simulink model "Lab3Part2B2"  (R2025b)
settings: Solver=VariableStepAuto  StartTime=0.0  StopTime=10.0  RelTol=1e-3
values from neighbouring files (symbols this model uses):
  A = [0 0 1 0 ... (first row only)    [Lab3Part2B1.m]
  B = [0 ... (first row only)    [Lab3Part2B1.m]
  K = place(A,B,desired_poles)    [Lab3Part2B1.m]
libraries: simulink_extras x3
settings Model: Creator=safiakhalil  LastModifiedBy=safiakhalil

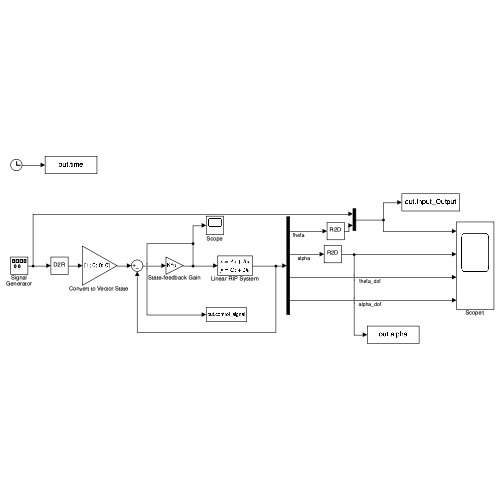
[thumbnail: Simulink's stored preview of the top-level diagram]
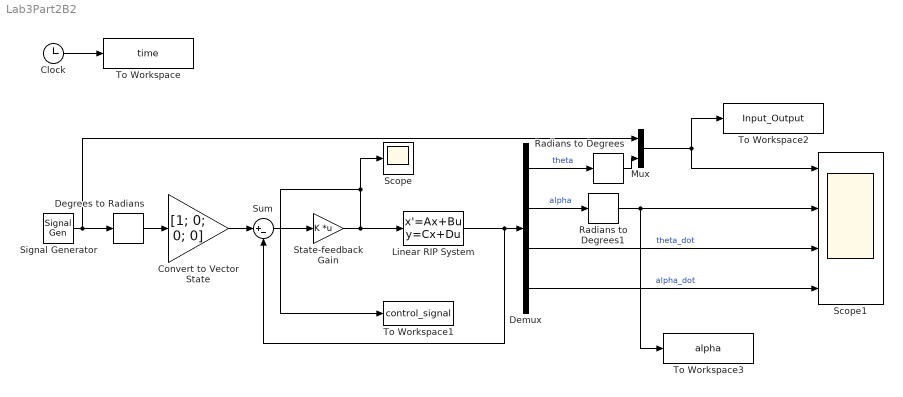
== system Lab3Part2B2 ==
  Clock : Clock
  "Convert to Vector State " : Gain  Gain=[1; 0; 0; 0]
  Degrees to Radians : simulink_extras/Transformations/Degrees to Radians
  Demux : Demux
  Linear RIP System : StateSpace  A=A  B=B  C=eye(4)  D=zeros(4, 1)  InitialCondition=0
  Mux : Mux  Inputs=2
  Radians to Degrees : simulink_extras/Transformations/Radians to Degrees
  Radians to Degrees1 : simulink_extras/Transformations/Radians to Degrees
  Scope : Scope
      settings: ActiveDisplayYMinimum=-0.48303961854114436  ActiveDisplayYMaximum=0.48467023948413279
  Scope1 : Scope  NumInputPorts=4
      settings: ActiveDisplayYMinimum=-1  ActiveDisplayYMaximum=1
  Signal Generator : SignalGenerator  WaveForm=square  Amplitude=20  Frequency=0.1
  State-feedback Gain : Gain  Gain=K  Multiplication=Matrix(K*u)
  Sum : Sum  Inputs=|+-
  To Workspace : ToWorkspace  VariableName=time  SampleTime=-1
  To Workspace1 : ToWorkspace  VariableName=control_signal  SampleTime=-1
  To Workspace2 : ToWorkspace  VariableName=Input_Output  SampleTime=-1
  To Workspace3 : ToWorkspace  VariableName=alpha  SampleTime=-1
  wires:
  Clock/1 -> To Workspace/1
  Linear RIP System/1 -> Demux/1, Sum/2
  Radians to Degrees/1 -> Mux/2
  Demux/1 -> Radians to Degrees/1  "theta"
  Demux/2 -> Radians to Degrees1/1  "alpha"
  Mux/1 -> Scope1/1, To Workspace2/1
  Radians to Degrees1/1 -> To Workspace3/1, Scope1/2
  Demux/4 -> Scope1/4  "alpha_dot"
  Demux/3 -> Scope1/3  "theta_dot"
  Signal Generator/1 -> Degrees to Radians/1, Mux/1
  Degrees to Radians/1 -> "Convert to Vector State "/1
  "Convert to Vector State "/1 -> Sum/1
  Sum/1 -> State-feedback Gain/1
  State-feedback Gain/1 -> To Workspace1/1, Scope/1, Linear RIP System/1
